simulink model "FifthOrdMdl"  (R2023b)
settings: Solver=ode5  StartTime=0.0  StopTime=50  FixedStep=1e-3  RelTol=1e-3
values from neighbouring files (symbols this model uses):
  A = [Kx1 Kx2; 0 -1/tau_theta]    [SecondOrderModel.m]    (also in SecondOrderModel_Final.m = [getAerodynamics(x0(1)*1/Ng,x0(2),v)/(J*x0(1)^2)-Dg/J 0)
  B = [0; 1/tau_theta]    [SecondOrderModel.m]    (also in SecondOrderModel_Final.m = [Dg*omega_0/(J*p*x0(2)); 1/tau_theta])
  C = diag([1 1])    [SecondOrderModel.m]    (also in SecondOrderModel_Final.m)
  Ds = 8*1e4    (= 80000)    [Parameters.m]
  Jg = 10    [Parameters.m]
  Jr = 90000    [Parameters.m]
  K = lqr(A,B,Q,R)    [SecondOrderModel_Final.m]
  Ks = 8*1e6    (= 8000000)    [Parameters.m]
  Ng = 24.6    [Parameters.m]
  omega_g0 = 105.62    [Parameters.m]
  omega_r0 = 4.29    [Parameters.m]
  tau_T = 0.1    [Parameters.m]
  tau_theta = 0.15    [Parameters.m]
  theta_max = 25    [Parameters.m]
  theta_min = -1    [Parameters.m]
  x0 = [1; 1]    [FifthOrderModel.m]    (also in SecondOrderModel.m = [omega_g0; u0]; SecondOrderModel_Final.m = [omega_g0; u0])
libraries: slpidlib x2, cstblocks x1
settings Model: Creator=Selim  LastModifiedBy=Selim

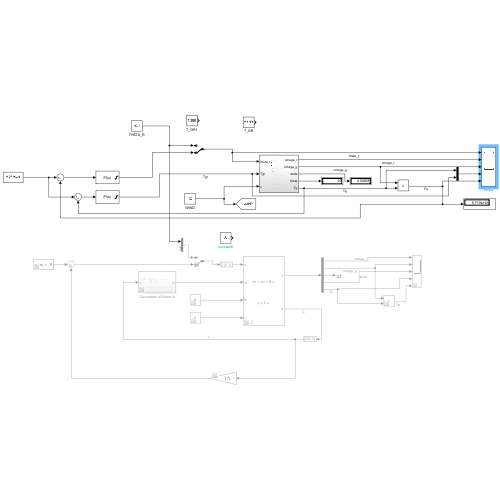
[thumbnail: Simulink's stored preview of the top-level diagram]
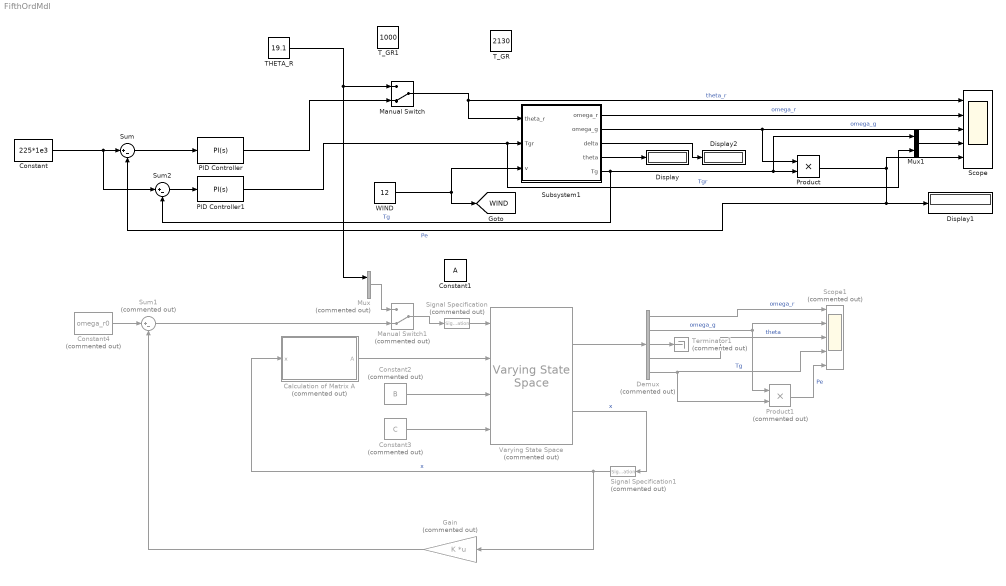
== system FifthOrdMdl ==
  Calculation of Matrix A : Subsystem  Commented=on
  Constant : Constant  Value=225*1e3
  Constant1 : Constant  Value=A
  Constant2 : Constant  Commented=on  Value=B
  Constant3 : Constant  Commented=on  Value=C
  Constant4 : Constant  Commented=on  Value=omega_r0
  Demux : Demux  Commented=on  Outputs=5
  Display : Display
  Display1 : Display
  Display2 : Display
  Gain : Gain  Commented=on  Gain=K  Multiplication=Matrix(K*u)
  Manual Switch : ManualSwitch  CurrentSetting=0
  Manual Switch1 : ManualSwitch  Commented=on  CurrentSetting=0
  Mux : Mux  Commented=on  Inputs=2
  Mux1 : Mux  Inputs=2
  PID Controller : slpidlib/PID Controller  Controller=PI  Form=Parallel  TimeDomain=Continuous-time  UseExternalTs=off  SampleTime=-1  IntegratorMethod=Forward Euler  FilterMethod=Forward Euler  ControllerParametersSource=internal  P=103.063598194959  I=163.792576247662  UseKiTs=off  D=0  N=100  UseFilter=on  TunerSelectOption=Transfer Function Based (PID Tuner App)  InitialConditionSource=internal  InitialConditionForIntegrator=0  InitialConditionForFilter=0  DifferentiatorICPrevScaledInput=0  ExternalReset=none  TrackingMode=off  Kt=1  LimitOutput=on  SatLimitsSource=internal  UpperSaturationLimit=theta_max  LowerSaturationLimit=theta_min  LinearizeAsGain=on  AntiWindupMode=clamping  Kb=1  LimitIntegrator=off  UpperIntegratorSaturationLimit=inf  LowerIntegratorSaturationLimit=-inf  POutMin=[]  POutMax=[]  IOutMin=[]  IOutMax=[]  DOutMin=[]  DOutMax=[]  NOutMin=[]  NOutMax=[]  SumOutMin=[]  SumOutMax=[]  SaturationOutMin=[]  SaturationOutMax=[]  PParamMin=[]  PParamMax=[]  IParamMin=[]  IParamMax=[]  DParamMin=[]  DParamMax=[]  NParamMin=[]  NParamMax=[]  KbParamMin=[]  KbParamMax=[]  KtParamMin=[]  KtParamMax=[]  KbOutMin=[]  KbOutMax=[]  KtOutMin=[]  KtOutMax=[]  IntegratorOutMin=[]  IntegratorOutMax=[]  FilterOutMin=[]  FilterOutMax=[]  SumI1OutMin=[]  SumI1OutMax=[]  SumI2OutMin=[]  SumI2OutMax=[]  SumI3OutMin=[]  SumI3OutMax=[]  SumI4OutMin=[]  SumI4OutMax=[]  SumDOutMin=[]  SumDOutMax=[]  DifferentiatorOutMin=[]  DifferentiatorOutMax=[]  FilterDiffOutCoefMin=[]  FilterDiffOutCoefMax=[]  ReciprocalOutMin=[]  ReciprocalOutMax=[]  SumDenOutMin=[]  SumDenOutMax=[]  SumNumOutMin=[]  SumNumOutMax=[]  DivideOutMin=[]  DivideOutMax=[]  UdiffTsProdOutMin=[]  UdiffTsProdOutMax=[]  NTsProdOutMin=[]  NTsProdOutMax=[]  UintegralTsProdOutMin=[]  UintegralTsProdOutMax=[]  UngainTsProdOutMin=[]  UngainTsProdOutMax=[]  ClampingZeroOutDataTypeStr=Inherit: Inherit via back propagation  ClampingZeroOutMin=[]  ClampingZeroOutMax=[]  FilterDenConstantOutDataTypeStr=Inherit: Inherit via back propagation  FilterDenConstantOutMin=[]  FilterDenConstantOutMax=[]  PCopyOutDataTypeStr=Inherit: Inherit via back propagation  PCopyOutMin=[]  PCopyOutMax=[]  NCopyOutDataTypeStr=Inherit: Inherit via back propagation  NCopyOutMin=[]  NCopyOutMax=[]  IntegratorContinuousStateAttributes=''  IntegratorStateMustResolveToSignalObject=off  IntegratorRTWStateStorageClass=Auto  FilterContinuousStateAttributes=''  FilterStateMustResolveToSignalObject=off  FilterRTWStateStorageClass=Auto  ParallelPVariant=InternalParameters  IdealPVariant=Disabled  IVariant=InternalParameters  DVariant=Disabled  IntegratorVariant=Continuous  SatVariant=Enabled  AWVariant=ContClampingParallel  PCopyVariant=Disabled  TRVariant=Disabled  FdbkBlocksVariant=Forward  IdealPFdbkVariant=Disabled  SatFdbkVariant=Disabled  DerivativeFilterVariant=Disabled  NVariant=Disabled  NCopyVariant=Disabled_SignalSpec  FilterICVariant=Disabled  IntegratorICVariant=InternalICs  ExternalResetVariant=Disabled  TRSumVariant=Passthrough  SumFdbkVariant=Disabled  SumVariant=Sum_PI  TsampFilterVariant=InternalTs  TsampNgainVariant=Passthrough  TsampIntegralVariant=Disabled_SignalSpec  ExternalSaturationOutDataTypeStr=Inherit: Same as second input
  PID Controller1 : slpidlib/PID Controller  Controller=PI  Form=Parallel  TimeDomain=Continuous-time  UseExternalTs=off  SampleTime=-1  IntegratorMethod=Forward Euler  FilterMethod=Forward Euler  ControllerParametersSource=internal  P=0  I=3.2399032238793  UseKiTs=off  D=0  N=100  UseFilter=on  TunerSelectOption=Transfer Function Based (PID Tuner App)  InitialConditionSource=internal  InitialConditionForIntegrator=0  InitialConditionForFilter=0  DifferentiatorICPrevScaledInput=0  ExternalReset=none  TrackingMode=off  Kt=1  LimitOutput=on  SatLimitsSource=internal  UpperSaturationLimit=2130  LowerSaturationLimit=-2130  LinearizeAsGain=on  AntiWindupMode=clamping  Kb=1  LimitIntegrator=off  UpperIntegratorSaturationLimit=inf  LowerIntegratorSaturationLimit=-inf  POutMin=[]  POutMax=[]  IOutMin=[]  IOutMax=[]  DOutMin=[]  DOutMax=[]  NOutMin=[]  NOutMax=[]  SumOutMin=[]  SumOutMax=[]  SaturationOutMin=[]  SaturationOutMax=[]  PParamMin=[]  PParamMax=[]  IParamMin=[]  IParamMax=[]  DParamMin=[]  DParamMax=[]  NParamMin=[]  NParamMax=[]  KbParamMin=[]  KbParamMax=[]  KtParamMin=[]  KtParamMax=[]  KbOutMin=[]  KbOutMax=[]  KtOutMin=[]  KtOutMax=[]  IntegratorOutMin=[]  IntegratorOutMax=[]  FilterOutMin=[]  FilterOutMax=[]  SumI1OutMin=[]  SumI1OutMax=[]  SumI2OutMin=[]  SumI2OutMax=[]  SumI3OutMin=[]  SumI3OutMax=[]  SumI4OutMin=[]  SumI4OutMax=[]  SumDOutMin=[]  SumDOutMax=[]  DifferentiatorOutMin=[]  DifferentiatorOutMax=[]  FilterDiffOutCoefMin=[]  FilterDiffOutCoefMax=[]  ReciprocalOutMin=[]  ReciprocalOutMax=[]  SumDenOutMin=[]  SumDenOutMax=[]  SumNumOutMin=[]  SumNumOutMax=[]  DivideOutMin=[]  DivideOutMax=[]  UdiffTsProdOutMin=[]  UdiffTsProdOutMax=[]  NTsProdOutMin=[]  NTsProdOutMax=[]  UintegralTsProdOutMin=[]  UintegralTsProdOutMax=[]  UngainTsProdOutMin=[]  UngainTsProdOutMax=[]  ClampingZeroOutDataTypeStr=Inherit: Inherit via back propagation  ClampingZeroOutMin=[]  ClampingZeroOutMax=[]  FilterDenConstantOutDataTypeStr=Inherit: Inherit via back propagation  FilterDenConstantOutMin=[]  FilterDenConstantOutMax=[]  PCopyOutDataTypeStr=Inherit: Inherit via back propagation  PCopyOutMin=[]  PCopyOutMax=[]  NCopyOutDataTypeStr=Inherit: Inherit via back propagation  NCopyOutMin=[]  NCopyOutMax=[]  IntegratorContinuousStateAttributes=''  IntegratorStateMustResolveToSignalObject=off  IntegratorRTWStateStorageClass=Auto  FilterContinuousStateAttributes=''  FilterStateMustResolveToSignalObject=off  FilterRTWStateStorageClass=Auto  ParallelPVariant=InternalParameters  IdealPVariant=Disabled  IVariant=InternalParameters  DVariant=Disabled  IntegratorVariant=Continuous  SatVariant=Enabled  AWVariant=ContClampingParallel  PCopyVariant=Disabled  TRVariant=Disabled  FdbkBlocksVariant=Forward  IdealPFdbkVariant=Disabled  SatFdbkVariant=Disabled  DerivativeFilterVariant=Disabled  NVariant=Disabled  NCopyVariant=Disabled_SignalSpec  FilterICVariant=Disabled  IntegratorICVariant=InternalICs  ExternalResetVariant=Disabled  TRSumVariant=Passthrough  SumFdbkVariant=Disabled  SumVariant=Sum_PI  TsampFilterVariant=InternalTs  TsampNgainVariant=Passthrough  TsampIntegralVariant=Disabled_SignalSpec  ExternalSaturationOutDataTypeStr=Inherit: Same as second input
  Product : Product
  Product1 : Product  Commented=on
  Scope : Scope  NumInputPorts=5
  Scope1 : Scope  Commented=on  NumInputPorts=5
  Signal Specification : SignalSpecification  Commented=on  Dimensions=[2 1]
  Signal Specification1 : SignalSpecification  Commented=on  Dimensions=[5 1]
  Subsystem1 : Subsystem
  Sum : Sum  Inputs=|+-
  Sum1 : Sum  Commented=on  Inputs=|+-
  Sum2 : Sum  Inputs=|+-
  THETA_R : Constant  Value=19.1
  T_GR : Constant  Value=2130
  T_GR1 : Constant  Value=1000
  Terminator1 : Terminator  Commented=on
  Varying State Space : cstblocks/Linear Parameter Varying/Varying State Space  Commented=on  x0=x0  xNames=''  OutputX=on  OutputDX=off  Feedthrough=off
  WIND : Constant  Value=12
  tag scope: WIND=global
  wires:
  WIND/1 -> [WIND], Subsystem1/3(v)
  THETA_R/1 -> Mux/1, Manual Switch/1
  Subsystem1/2(omega_g) -> Product/1, Scope/3  "omega_g"
  Subsystem1/5(Tg) -> Sum2/2, Mux1/1, Product/2  "Tg"
  Product/1 -> Display1/1, Sum/2, Scope/5  "Pe"
  Subsystem1/1(omega_r) -> Scope/2  "omega_r"
  Subsystem1/4(theta) -> Display/1
  Subsystem1/3(delta) -> Display2/1
  Sum/1 -> PID Controller/1
  PID Controller/1 -> Manual Switch/2
  Constant/1 -> Sum2/1, Sum/1
  Manual Switch/1 -> Scope/1, Subsystem1/1(theta_r)  "theta_r"
  Mux/1 -> Manual Switch1/1
  Signal Specification/1 -> Varying State Space/1
  Constant2/1 -> Varying State Space/3
  Constant3/1 -> Varying State Space/4
  Varying State Space/1 -> Demux/1
  Varying State Space/2 -> Signal Specification1/1  "x"
  Demux/1 -> Scope1/1  "omega_r"
  Demux/2 -> Product1/1, Scope1/2  "omega_g"
  Demux/3 -> Terminator1/1
  Demux/4 -> Scope1/3  "theta"
  Demux/5 -> Scope1/4, Product1/2  "Tg"
  Signal Specification1/1 -> Gain/1, Calculation of Matrix A/1(x)  "x"
  Calculation of Matrix A/1(A) -> Varying State Space/2
  Product1/1 -> Scope1/5  "Pe"
  Manual Switch1/1 -> Signal Specification/1
  Gain/1 -> Sum1/2
  Sum1/1 -> Manual Switch1/2
  Constant4/1 -> Sum1/1
  Sum2/1 -> PID Controller1/1
  PID Controller1/1 -> Mux1/2, Subsystem1/2(Tgr)  "Tgr"
  Mux1/1 -> Scope/4

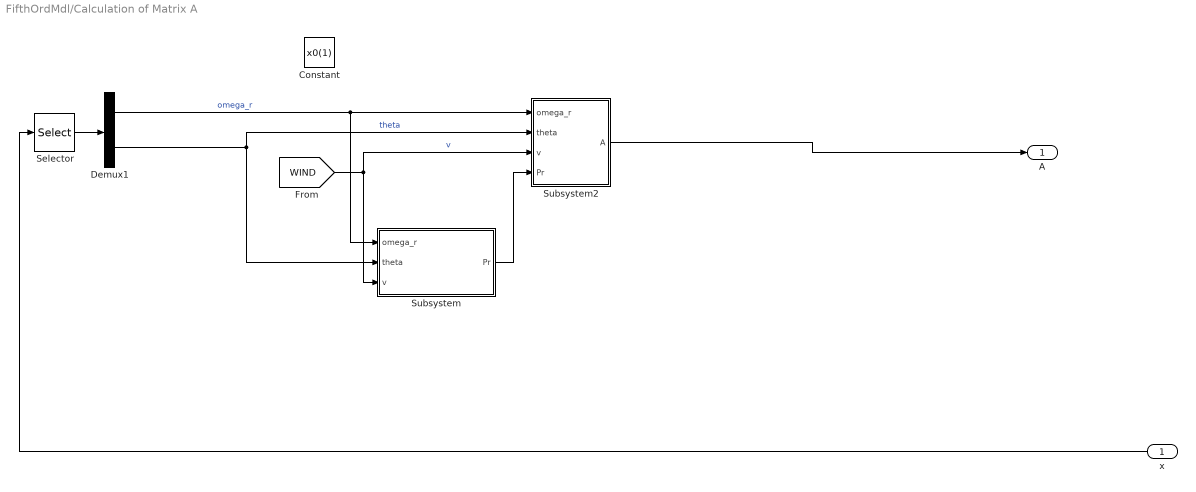
== system FifthOrdMdl/Calculation of Matrix A ==
  x : Inport
  Constant : Constant  Value=x0(1)
  Demux1 : Demux  Outputs=2
  Selector : Selector  InputPortWidth=5  IndexOptions=Index vector (dialog)  Indices=[1 4]  OutputSizes=1
  Subsystem : Subsystem
  Subsystem2 : Subsystem
  A : Outport
  wires:
  Demux1/1 -> Subsystem/1(omega_r), Subsystem2/1(omega_r)  "omega_r"
  x/1 -> Selector/1
  Subsystem/1(Pr) -> Subsystem2/4(Pr)
  Demux1/2 -> Subsystem2/2(theta), Subsystem/2(theta)  "theta"
  Selector/1 -> Demux1/1
  [WIND] -> Subsystem2/3(v), Subsystem/3(v)  "v"
  Subsystem2/1(A) -> A/1

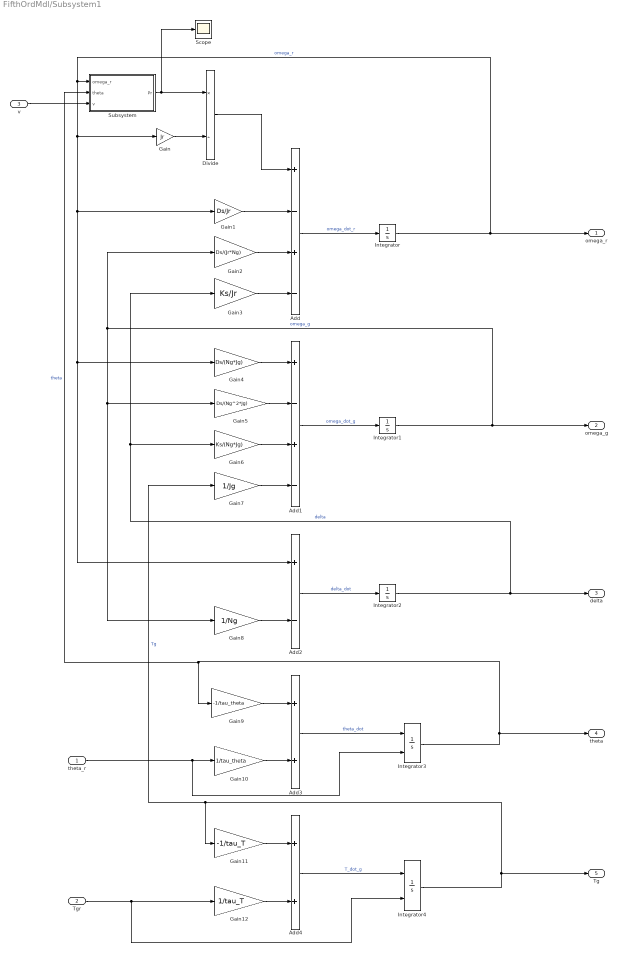
== system FifthOrdMdl/Subsystem1 ==
  theta_r : Inport
  Tgr : Inport  Port=2
  v : Inport  Port=3
  Add : Sum  Inputs=+-+-
  Add1 : Sum  Inputs=+-+-
  Add2 : Sum  Inputs=+-
  Add3 : Sum
  Add4 : Sum
  Divide : Product  Inputs=*/
  Gain : Gain  Gain=Jr
  Gain1 : Gain  Gain=Ds/Jr
  Gain10 : Gain  Gain=1/tau_theta
  Gain11 : Gain  Gain=-1/tau_T
  Gain12 : Gain  Gain=1/tau_T
  Gain2 : Gain  Gain=Ds/(Jr*Ng)
  Gain3 : Gain  Gain=Ks/Jr
  Gain4 : Gain  Gain=Ds/(Ng*Jg)
  Gain5 : Gain  Gain=Ds/(Ng^2*Jg)
  Gain6 : Gain  Gain=Ks/(Ng*Jg)
  Gain7 : Gain  Gain=1/Jg
  Gain8 : Gain  Gain=1/Ng
  Gain9 : Gain  Gain=-1/tau_theta
  Integrator : Integrator  InitialCondition=omega_r0
  Integrator1 : Integrator  InitialCondition=omega_g0
  Integrator2 : Integrator  InitialCondition=6.55*1e-3
  Integrator3 : Integrator  InitialConditionSource=external
  Integrator4 : Integrator  InitialConditionSource=external  InitialCondition=2130
  Scope : Scope
  Subsystem : Subsystem
  omega_r : Outport
  omega_g : Outport  Port=2
  delta : Outport  Port=3
  theta : Outport  Port=4
  Tg : Outport  Port=5
  wires:
  Integrator2/1 -> delta/1, Gain6/1, Gain3/1  "delta"
  Integrator1/1 -> omega_g/1, Gain2/1, Gain8/1, Gain5/1  "omega_g"
  Add3/1 -> Integrator3/1  "theta_dot"
  Gain5/1 -> Add1/2
  Gain4/1 -> Add1/1
  Integrator3/1 -> theta/1, Subsystem/2(theta), Gain9/1  "theta"
  Gain11/1 -> Add4/1
  Integrator4/1 -> Tg/1, Gain7/1, Gain11/1  "Tg"
  Gain/1 -> Divide/2
  Integrator/1 -> omega_r/1, Add2/1, Gain4/1, Gain1/1, Gain/1, Subsystem/1(omega_r)  "omega_r"
  theta_r/1 -> Integrator3/2, Gain10/1
  Gain10/1 -> Add3/2
  v/1 -> Subsystem/3(v)
  Subsystem/1(Pr) -> Scope/1, Divide/1
  Add/1 -> Integrator/1  "omega_dot_r"
  Gain12/1 -> Add4/2
  Gain3/1 -> Add/4
  Add4/1 -> Integrator4/1  "T_dot_g"
  Gain6/1 -> Add1/3
  Gain2/1 -> Add/3
  Gain7/1 -> Add1/4
  Gain1/1 -> Add/2
  Divide/1 -> Add/1
  Add1/1 -> Integrator1/1  "omega_dot_g"
  Gain9/1 -> Add3/1
  Add2/1 -> Integrator2/1  "delta_dot"
  Gain8/1 -> Add2/2
  Tgr/1 -> Integrator4/2, Gain12/1

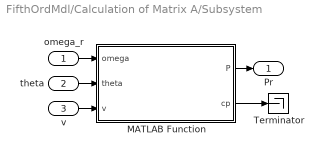
== system FifthOrdMdl/Calculation of Matrix A/Subsystem ==
  omega_r : Inport
  theta : Inport  Port=2
  v : Inport  Port=3
  MATLAB Function : MATLAB Function  TreatAsAtomicUnit=on
  Terminator : Terminator
  Pr : Outport
  wires:
  theta/1 -> MATLAB Function/2(theta)
  MATLAB Function/2(cp) -> Terminator/1
  omega_r/1 -> MATLAB Function/1(omega)
  v/1 -> MATLAB Function/3(v)
  MATLAB Function/1(P) -> Pr/1

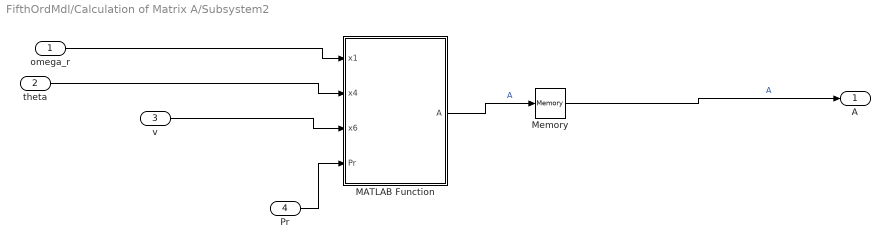
== system FifthOrdMdl/Calculation of Matrix A/Subsystem2 ==
  omega_r : Inport
  theta : Inport  Port=2
  v : Inport  Port=3
  Pr : Inport  Port=4
  MATLAB Function : MATLAB Function  TreatAsAtomicUnit=on
  Memory : Memory  InitialCondition=A
  A : Outport
  wires:
  MATLAB Function/1(A) -> Memory/1  "A"
  Memory/1 -> A/1  "A"
  v/1 -> MATLAB Function/3(x6)
  theta/1 -> MATLAB Function/2(x4)
  Pr/1 -> MATLAB Function/4(Pr)
  omega_r/1 -> MATLAB Function/1(x1)

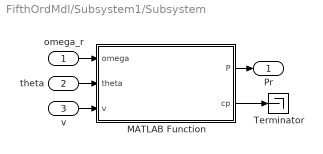
== system FifthOrdMdl/Subsystem1/Subsystem ==
  omega_r : Inport
  theta : Inport  Port=2
  v : Inport  Port=3
  MATLAB Function : MATLAB Function  TreatAsAtomicUnit=on
  Terminator : Terminator
  Pr : Outport
  wires:
  theta/1 -> MATLAB Function/2(theta)
  MATLAB Function/2(cp) -> Terminator/1
  omega_r/1 -> MATLAB Function/1(omega)
  v/1 -> MATLAB Function/3(v)
  MATLAB Function/1(P) -> Pr/1

== matlab function FifthOrdMdl/Calculation of Matrix A/Subsystem2/MATLAB Function ==
  data: x1 input; A output; x4 input; x6 input; Pr input; Jr parameter; Ds parameter; Ng parameter; tau_theta parameter; tau_T parameter; Ks parameter; Jg parameter
function A  = getMatrixA(x1,x4,x6,Pr,Jr, Ds, Ng, tau_theta, tau_T, Ks, Jg)

F1 = - (23340273*x6^2*pi*exp(7/(160*((27*x4^3)/8 + 1)) - 25/(2*((3*x4)/25 + (29*x1)/(2*x6)))))/(500*((3*x4)/25 + (29*x1)/(2*x6))^2) - (365835*x6^2*pi*exp(7/(160*((27*x4^3)/8 + 1)) - 25/(2*((3*x4)/25 + (29*x1)/(2*x6))))*((33*x4)/250 - 638/(25*((3*x4)/25 + (29*x1)/(2*x6))) + 2233/(25000*((27*x4^3)/8 + 1)) + 11/10))/(16*((3*x4)/25 + (29*x1)/(2*x6))^2);
F4 = (2523*x6^3*pi*exp(7/(160*((27*x4^3)/8 + 1)) - 25/(2*((3*x4)/25 + (29*x1)/(2*x6))))*((567*x4^2)/(1280*((27*x4^3)/8 + 1)^2) - 3/(2*((3*x4)/25 + (29*x1)/(2*x6))^2))*((33*x4)/250 - 638/(25*((3*x4)/25 + (29*x1)/(2*x6))) + 2233/(25000*((27*x4^3)/8 + 1)) + 11/10))/20 - (2523*x6^3*pi*exp(7/(160*((27*x4^3)/8 + 1)) - 25/(2*((3*x4)/25 + (29*x1)/(2*x6))))*(1914/(625*((3*x4)/25 + (29*x1)/(2*x6))^2) - (180873*x4^2)/(200000*((27*x4^3)/8 + 1)^2) + 33/250))/20;

K11 = F1/(x1*Jr) - Pr/((x1^2)*Jr) - Ds/Jr;
K14 = F4/(x1*Jr);

A = [K11 Ds/(Jr*Ng) -Ks/Jr K14 0;
     Ds/(Jg*Ng) -Ds/(Ng^2*Jg) Ks/(Jg*Ng) 0 -1/Jg;
     1 -1/Ng 0 0 0;
     0 0 0 -1/tau_theta 0;
     0 0 0 0 -1/tau_T];

== matlab function FifthOrdMdl/Subsystem1/Subsystem/MATLAB Function ==
  data: omega input; P output; theta input; v input; cp output
function [P,cp] = getAerodynamics(omega,theta,v)

R = 14.5;
rho = 1.2;

lambda = v/(R*omega);
lambda_t = 1/(1/(lambda^-1 + 0.12*theta) - 0.0035/((1.5*theta)^3 + 1));

cp = 0.22*(116/lambda_t - 0.6*theta - 5)*exp(-12.5/lambda_t);

P = 1/2*rho*pi*(R^2)*(v^3)*cp;

== matlab function FifthOrdMdl/Calculation of Matrix A/Subsystem/MATLAB Function ==
  data: omega input; P output; theta input; v input; cp output
function [P,cp] = getAerodynamics(omega,theta,v)

R = 14.5;
rho = 1.2;

lambda = v/(R*omega);
lambda_t = 1/(1/(lambda^-1 + 0.12*theta) - 0.0035/((1.5*theta)^3 + 1));

cp = 0.22*(116/lambda_t - 0.6*theta - 5)*exp(-12.5/lambda_t);

P = 1/2*rho*pi*(R^2)*(v^3)*cp;
